simulink model "couple_dmp_test"  (R2020b)
settings: Solver=ode8  StartTime=0.0  StopTime=10.0  FixedStep=0.005  RelTol=1e-3
values from neighbouring files (symbols this model uses):
  Am = [1 8 10]    [my_config_1213.mat]    (also in my_config_1219.mat)
  Bm = [1 10]    [my_config_1213.mat]    (also in my_config_1219.mat)
  cc = [1 0.92774349 0.86070798 0.79851622 0.74081822 0.68728928 0.63762815 0.59155536 0.54881164 0.50915642 0.47236655 0.43823499 ... (41 elements, 1x41)]    [my_config_1213.mat]    (also in my_config_1219.mat)
  D = [64.807 64.807 64.807]    [my_config_1213.mat]    (also in my_config_1219.mat)
  g1 = [-1 0 1]    [my_config_1213.mat]
  g2 = [-1 0.6 1]    [my_config_1213.mat]
  gamma1 = 1.2    [my_config_1213.mat]    (also in my_config_1219.mat)
  gamma2 = 0.5    [my_config_1213.mat]    (also in my_config_1219.mat)
  K = [1050 1050 1050]    [my_config_1213.mat]    (also in my_config_1219.mat; my_config_1224.mat)
  left_0 = [0 0 0]    [my_config_1219.mat]
  m1 = 1    [my_config_1213.mat]    (also in my_config_1219.mat; my_config_1224.mat)
  m2 = 1    [my_config_1213.mat]    (also in my_config_1219.mat; my_config_1224.mat)
  right_0 = [0 0.6 0]    [my_config_1213.mat]    (also in my_config_1219.mat)
  tau1 = 3    [my_config_1213.mat]    (also in my_config_1219.mat)
  weight = [0.0266866854 0.00199886353 0 0.185908993 0.0191898792 0 0.285018336 0.0372844837 0 0.420259935 0.0646488362 0 ... (123 elements, 3x41)]    [my_config_1213.mat]    (also in my_config_1219.mat)
  width = [191.53405062 222.53081866 258.54392519 300.38518553 348.99779456 405.47758835 471.09774681 547.33749391 635.91544276 738.82833688 858.39606128 997.31393782 ... (41 elements, 1x41)]    [my_config_1213.mat]    (also in my_config_1219.mat)
  x1_0 = [0 0.2 0]    [my_config_1213.mat]    (also in my_config_1219.mat; my_config_1224.mat)
  x2_0 = [0 0.4 0]    [my_config_1213.mat]    (also in my_config_1219.mat; my_config_1224.mat)
undefined symbols (not defined in the file or in its folder): b1, b2, b3, k1, k2, k3
settings Model: Creator=10788  LastModifiedBy=10788
settings OptimizationCC: DefaultParameterBehavior=Inlined  UseDivisionForNetSlopeComputation=on  GainParamInheritBuiltInType=on  UseFloatMulNetSlope=on  InlineInvariantSignals=on  PassReuseOutputArgsAs=Individual arguments  ZeroExternalMemoryAtStartup=off  ZeroInternalMemoryAtStartup=off  NoFixptDivByZeroProtection=on  EfficientFloat2IntCast=on  LifeSpan=1  OptimizeBlockOrder=speed  DifferentSizesBufferReuse=on  EfficientTunableParamExpr=on
settings DebuggingCC: ParameterTunabilityLossMsg=error
settings HardwareCC: ProdLongLongMode=on
settings SFSimCC: MATLABDynamicMemAlloc=off  SimTargetLang=C++
settings RTWCC: Description=Embedded Coder  SystemTargetFile=ert.tlc  TemplateMakefile=ert_default_tmf  GenerateReport=on  LaunchReport=on  TargetLang=C++
settings CodeAppCC: ForceParamTrailComments=on  IgnoreCustomStorageClasses=off  OperatorAnnotations=on  SimulinkDataObjDesc=on  SFDataObjDesc=on  CustomSymbolStrGlobalVar=rt$N$M  CustomSymbolStrType=$N$M  CustomSymbolStrFcn=$N$M$F  CustomSymbolStrMacro=$N$M  InsertBlockDesc=on
settings ERTTargetCC: TargetLangStandard=C++03 (ISO)  GenerateSampleERTMain=on  IncludeMdlTerminateFcn=off  CombineSignalStateStructs=on  CodeInterfacePackaging=C++ class  SupportComplex=off  SupportContinuousTime=on  SupportNonInlinedSFcns=on  InlinedParameterPlacement=NonHierarchical  RootIOFormat=Structure reference  ERTCustomFileTemplate=example_file_process.tlc  ERTFilePackagingFormat=CompactWithDataFile

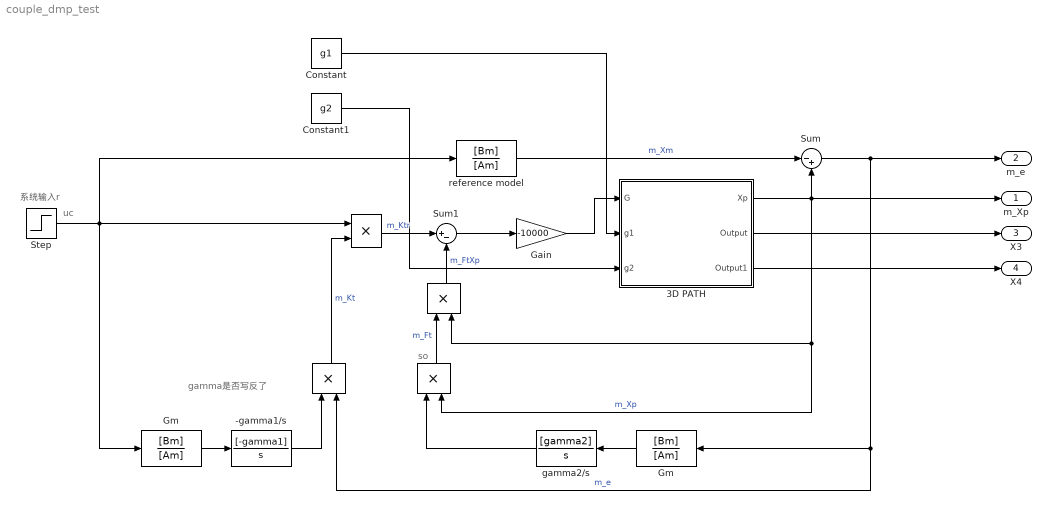
== system couple_dmp_test ==
  note: so
  note: gamma是否写反了
  note: uc
  note: 系统输入r
  " " : Product
  " " : Product
  "  " : Product
  "     " : Product
  -gamma1/s : TransferFcn  Numerator=[-gamma1]  Denominator=[1 0]
  3D PATH : Subsystem
  Constant : Constant  Value=g1
  Constant1 : Constant  Value=g2
  Gain : Gain  Gain=-10000
  "Gm " : TransferFcn  Numerator=[Bm]  Denominator=[Am]
  "Gm  " : TransferFcn  Numerator=[Bm]  Denominator=[Am]
  Step : Step  Time=0  After=0.2  SampleTime=0
  Sum : Sum  Inputs=|-+
  Sum1 : Sum  Inputs=|+-
  gamma2/s : TransferFcn  Numerator=[gamma2]  Denominator=[1 0]
  reference model : TransferFcn  Numerator=[Bm]  Denominator=[Am]
  m_Xp : Outport
  m_e : Outport  Port=2
  X3 : Outport  Port=3
  X4 : Outport  Port=4
  wires:
  "  "/1 -> " "/1  "m_Ft"
  reference model/1 -> Sum/1  "m_Xm"
  gamma2/s/1 -> "  "/1
  "     "/1 -> Sum1/1  "m_Ktr"
  3D PATH/1(Xp) -> "  "/2, " "/2, m_Xp/1, Sum/2  "m_Xp"
  " "/1 -> "     "/2  "m_Kt"
  -gamma1/s/1 -> " "/1
  Gain/1 -> 3D PATH/1(G)
  "Gm  "/1 -> -gamma1/s/1
  Sum1/1 -> Gain/1
  "Gm "/1 -> gamma2/s/1
  Sum/1 -> m_e/1, "Gm "/1, " "/2  "m_e"
  " "/1 -> Sum1/2  "m_FtXp"
  Step/1 -> "Gm  "/1, reference model/1, "     "/1
  3D PATH/2(Output) -> X3/1
  3D PATH/3(Output1) -> X4/1
  Constant/1 -> 3D PATH/2(g1)
  Constant1/1 -> 3D PATH/3(g2)

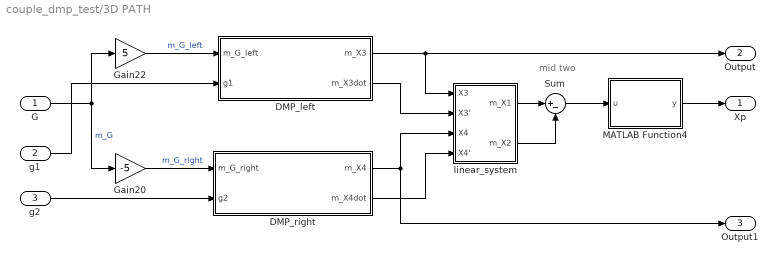
== system couple_dmp_test/3D PATH ==
  note: mid two
  G : Inport
  g1 : Inport  Port=2
  g2 : Inport  Port=3
  DMP_left : Subsystem
  DMP_right : Subsystem
  Gain20 : Gain  Gain=-5
  Gain22 : Gain  Gain=5
  MATLAB Function4 : MATLAB Function  TreatAsAtomicUnit=on
  Sum : Sum  Inputs=|+-
  linear_system : Subsystem
  Xp : Outport
  Output : Outport  Port=2
  Output1 : Outport  Port=3
  wires:
  G/1 -> Gain22/1, Gain20/1  "m_G"
  Sum/1 -> MATLAB Function4/1(u)
  MATLAB Function4/1(y) -> Xp/1
  Gain22/1 -> DMP_left/1(m_G_left)  "m_G_left"
  Gain20/1 -> DMP_right/1(m_G_right)  "m_G_right"
  DMP_left/1(m_X3) -> linear_system/1(X3), Output/1
  DMP_left/2(m_X3dot) -> linear_system/2(X3')
  DMP_right/1(m_X4) -> Output1/1, linear_system/3(X4)
  DMP_right/2(m_X4dot) -> linear_system/4(X4')
  linear_system/1(m_X1) -> Sum/1
  linear_system/2(m_X2) -> Sum/2
  g1/1 -> DMP_left/2(g1)
  g2/1 -> DMP_right/2(g2)

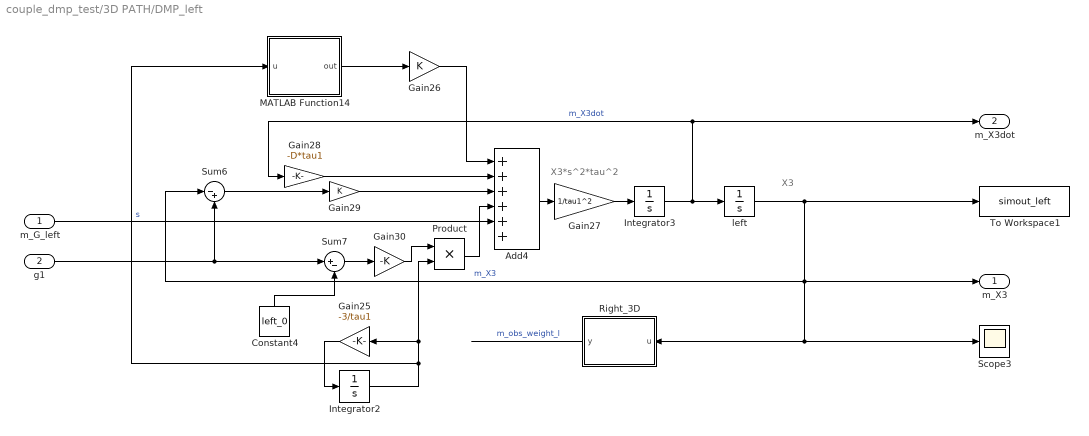
== system couple_dmp_test/3D PATH/DMP_left ==
  note: X3*s^2*tau^2
  note: X3
  m_G_left : Inport
  g1 : Inport  Port=2
  Add4 : Sum  Inputs=++++++
  Constant4 : Constant  Value=left_0
  Gain25 : Gain  Gain=-3/tau1
  Gain26 : Gain  Gain=K
  Gain27 : Gain  Gain=1/tau1^2
  Gain28 : Gain  Gain=-D*tau1
  Gain29 : Gain  Gain=K
  Gain30 : Gain  Gain=-K
  Integrator2 : Integrator  InitialCondition=1
  Integrator3 : Integrator
  MATLAB Function14 : MATLAB Function  TreatAsAtomicUnit=on
  Product : Product
  Right_3D : MATLAB Function  TreatAsAtomicUnit=on
  Scope3 : Scope
  Sum6 : Sum  Inputs=|-+
  Sum7 : Sum  Inputs=|+-
  To Workspace1 : ToWorkspace  VariableName=simout_left  SaveFormat=Timeseries  SampleTime=-1
  left : Integrator  InitialCondition=left_0
  m_X3 : Outport
  m_X3dot : Outport  Port=2
  wires:
  Gain26/1 -> Add4/1
  MATLAB Function14/1(out) -> Gain26/1
  Integrator2/1 -> MATLAB Function14/1(u), Gain25/1, Product/2  "s"
  Sum7/1 -> Gain30/1
  Gain29/1 -> Add4/3
  Gain25/1 -> Integrator2/1
  Gain28/1 -> Add4/2
  Product/1 -> Add4/4
  Gain27/1 -> Integrator3/1
  Sum6/1 -> Gain29/1
  Constant4/1 -> Sum7/2
  Add4/1 -> Gain27/1
  Integrator3/1 -> left/1, m_X3dot/1, Gain28/1  "m_X3dot"
  g1/1 -> Sum7/1, Sum6/2
  left/1 -> Sum6/1, m_X3/1, Right_3D/1(u), Scope3/1, To Workspace1/1  "m_X3"
  Gain30/1 -> Product/1
  m_G_left/1 -> Add4/5
  Right_3D/1(y) -> ?  "m_obs_weight_l"

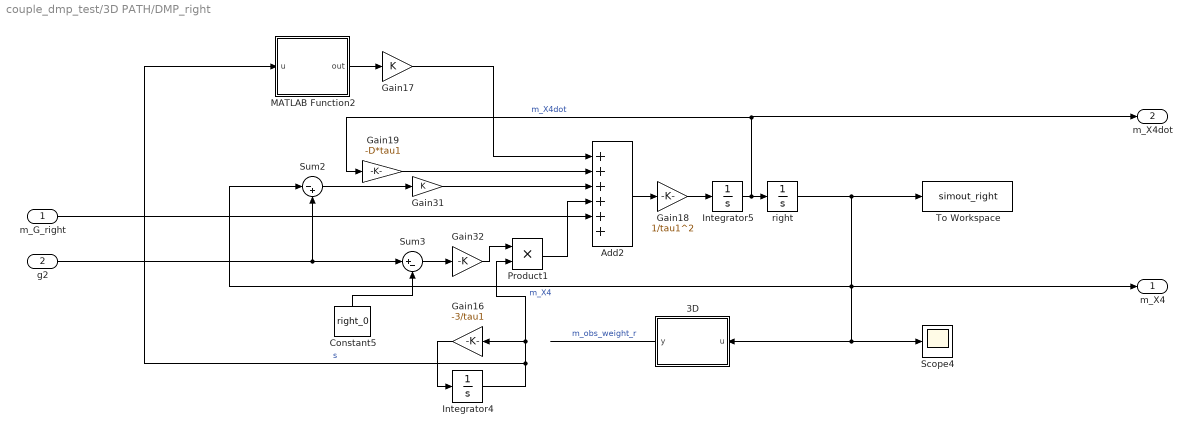
== system couple_dmp_test/3D PATH/DMP_right ==
  m_G_right : Inport
  g2 : Inport  Port=2
  3D : MATLAB Function  TreatAsAtomicUnit=on
  Add2 : Sum  Inputs=++++++
  Constant5 : Constant  Value=right_0
  Gain16 : Gain  Gain=-3/tau1
  Gain17 : Gain  Gain=K
  Gain18 : Gain  Gain=1/tau1^2
  Gain19 : Gain  Gain=-D*tau1
  Gain31 : Gain  Gain=K
  Gain32 : Gain  Gain=-K
  Integrator4 : Integrator  InitialCondition=1
  Integrator5 : Integrator
  MATLAB Function2 : MATLAB Function  TreatAsAtomicUnit=on
  Product1 : Product
  Scope4 : Scope
  Sum2 : Sum  Inputs=|-+
  Sum3 : Sum  Inputs=|+-
  To Workspace : ToWorkspace  VariableName=simout_right  SaveFormat=Timeseries  SampleTime=-1
  right : Integrator  InitialCondition=right_0
  m_X4 : Outport
  m_X4dot : Outport  Port=2
  wires:
  Gain31/1 -> Add2/3
  right/1 -> Sum2/1, m_X4/1, 3D/1(u), Scope4/1, To Workspace/1  "m_X4"
  MATLAB Function2/1(out) -> Gain17/1
  Gain16/1 -> Integrator4/1
  Integrator5/1 -> m_X4dot/1, Gain19/1, right/1  "m_X4dot"
  Sum2/1 -> Gain31/1
  Gain19/1 -> Add2/2
  Constant5/1 -> Sum3/2
  Product1/1 -> Add2/4
  Gain17/1 -> Add2/1
  Integrator4/1 -> Product1/2, Gain16/1, MATLAB Function2/1(u)  "s"
  Sum3/1 -> Gain32/1
  Gain18/1 -> Integrator5/1
  g2/1 -> Sum3/1, Sum2/2
  Add2/1 -> Gain18/1
  Gain32/1 -> Product1/1
  m_G_right/1 -> Add2/5
  3D/1(y) -> ?  "m_obs_weight_r"

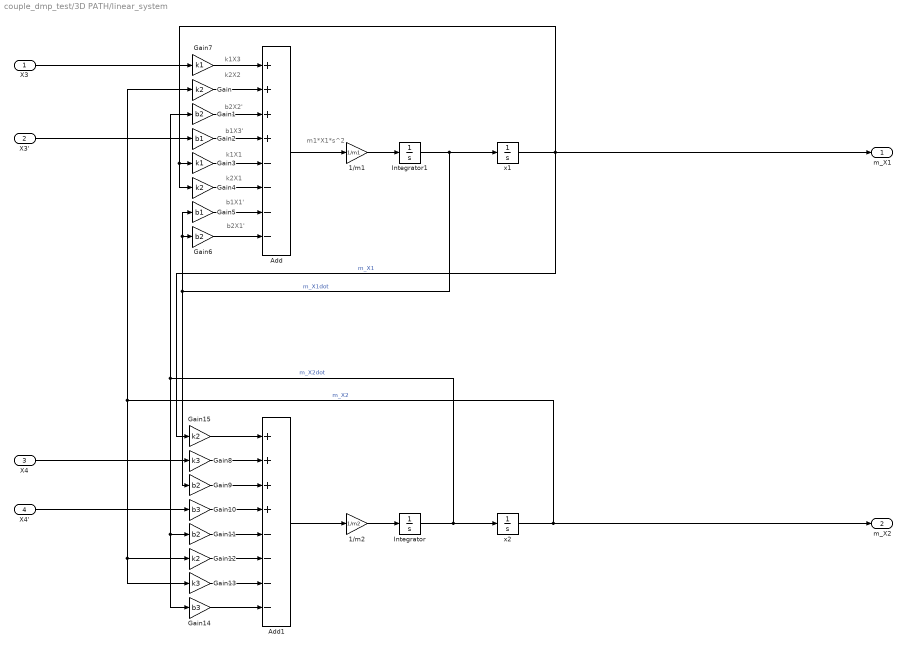
== system couple_dmp_test/3D PATH/linear_system ==
  note: m1*X1*s^2
  note: k1X3
  note: k2X2
  note: b2X2'
  note: b1X3'
  note: k1X1
  note: k2X1
  note: b1X1'
  note: b2X1'
  X3 : Inport
  X3' : Inport  Port=2
  X4 : Inport  Port=3
  X4' : Inport  Port=4
  1/m1 : Gain  Gain=1/m1
  1/m2 : Gain  Gain=1/m2
  Add : Sum  Inputs=++++----
  Add1 : Sum  Inputs=++++----
  Gain{,4,12,15} (4 alike) : Gain  Gain=k2
  Gain{1,6,9,11} (4 alike) : Gain  Gain=b2
  Gain10 : Gain  Gain=b3
  Gain13 : Gain  Gain=k3
  Gain14 : Gain  Gain=b3
  Gain2 : Gain  Gain=b1
  Gain3 : Gain  Gain=k1
  Gain5 : Gain  Gain=b1
  Gain7 : Gain  Gain=k1
  Gain8 : Gain  Gain=k3
  Integrator : Integrator
  Integrator1 : Integrator
  x1 : Integrator  InitialCondition=x1_0
  x2 : Integrator  InitialCondition=x2_0
  m_X1 : Outport
  m_X2 : Outport  Port=2
  wires:
  x1/1 -> Gain15/1, m_X1/1, Gain4/1, Gain3/1  "m_X1"
  Gain7/1 -> Add/1
  Gain3/1 -> Add/5
  1/m1/1 -> Integrator1/1
  Add1/1 -> 1/m2/1
  Gain2/1 -> Add/4
  Gain5/1 -> Add/7
  Gain4/1 -> Add/6
  Gain10/1 -> Add1/4
  X3/1 -> Gain7/1
  Gain6/1 -> Add/8
  Gain1/1 -> Add/3
  Gain15/1 -> Add1/1
  Integrator1/1 -> x1/1, Gain9/1, Gain5/1, Gain6/1  "m_X1dot"
  1/m2/1 -> Integrator/1
  x2/1 -> m_X2/1, Gain/1, Gain13/1, Gain12/1  "m_X2"
  Integrator/1 -> x2/1, Gain1/1, Gain14/1, Gain11/1  "m_X2dot"
  X3'/1 -> Gain2/1
  Add/1 -> 1/m1/1
  Gain/1 -> Add/2
  Gain14/1 -> Add1/8
  Gain13/1 -> Add1/7
  Gain8/1 -> Add1/2
  Gain11/1 -> Add1/5
  X4'/1 -> Gain10/1
  Gain9/1 -> Add1/3
  Gain12/1 -> Add1/6
  X4/1 -> Gain8/1

== matlab function couple_dmp_test/3D PATH/DMP_right/3D ==
  data: u input; y output
function y = fcn(u)

n_dim=3;
n_obt=2;
phi=zeros(n_dim,1);     % 3行1列
phi_tal=zeros(n_dim,1); % 2行1列

% 障碍物1
x_c_1 = 0.2;
y_c_1 = 0.8;
z_c_1 = 0.4;
a_1 = .1;
b_1 = .2;
c_1 = .1;

% 障碍物2
x_c_2 = -0.4;
y_c_2 = 1.2;
z_c_2 = 0.8;
a_2 = 0.15;
b_2 = 0.15;
c_2 = .2;

center=[x_c_1 y_c_1 z_c_1;
    x_c_2 y_c_2 z_c_2
];
axis=[a_1 b_1 c_1;
    a_2 b_2 c_2
];

% center=center(:,[2 1]);
% axis=axis(:,[2 1]);

%%%%%%%%%%%%%

for j=1:n_obt % 障碍物数量
    K = 0;
    for i = 1:n_dim % 坐标维度
        K =K+( (u(i) - center(j,i)) / axis(j,i)) ^2;
    end
    K = K - 1;

    for i = 1:n_dim
        phi(i) = (u(i) - center(j,i)) / axis(j,i) ^2;
    end

    phi = phi * ( exp(-K)) * (1 / K + 1 / K / K) * 2;
    phi_tal=phi_tal+phi;
end

y = phi_tal;

== matlab function couple_dmp_test/3D PATH/DMP_left/MATLAB Function14 ==
  data: u input; out output; width parameter; weight parameter; cc parameter
function out = fcn(u, width, weight, cc)


% if(u>2.5)
%     y=1;
% elseif(u>=0&&u<=2.5)
%     y=0;
% else
%         y=-1;
% end


tem=exp(-width.*(u-cc).^2)';
y=(weight*tem*u)/sum(tem) ;

out = y;

== matlab function couple_dmp_test/3D PATH/DMP_right/MATLAB Function2 ==
  data: u input; out output; width parameter; weight parameter; cc parameter
function out = fcn(u, width, weight, cc)


% if(u>2.5)
%     y=1;
% elseif(u>=0&&u<=2.5)
%     y=0;
% else
%         y=-1;
% end


tem=exp(-width.*(u-cc).^2)';
y=(weight*tem*u)/sum(tem) ;

out = y;

== matlab function couple_dmp_test/3D PATH/MATLAB Function4 ==
  data: u input; y output
function y = fcn(u)

y = norm(u);

== matlab function couple_dmp_test/3D PATH/DMP_left/Right_3D ==
  data: u input; y output
function y = fcn(u)

n_dim=3;
n_obt=1;
phi=zeros(n_dim,1);
phi_tal=zeros(n_dim,1);

x_c_1 = 0.15;
y_c_1 = 0.2;
z_c_1 = 0.4;
a_1 = .1;
b_1 = .1;
c_1 = .1;

x_c_2 = -0.4;
y_c_2 = 1.1;
z_c_2 = 0.8;
a_2 = 0.15;
b_2 = 0.15;
c_2 = .2;

% center=[x_c_1 y_c_1;
%     x_c_2 y_c_2];
% axis=[a_1 b_1;
%     a_2 b_2];

center=[x_c_1 y_c_1 z_c_1;
    x_c_2 y_c_2 z_c_2
];
axis=[a_1 b_1 c_1;
    a_2 b_2 c_2
];

% center=center(:,[2 1]);
% axis=axis(:,[2 1]);

%%%%%%%%%%%%%

for j=1:n_obt
    
    
    K = 0;
for i = 1:n_dim
    
    K =K+( (u(i) - center(j,i)) / axis(j,i)) ^2;
    
end
K = K - 1;

for i = 1:n_dim
    phi(i) = (u(i) - center(j,i)) / axis(j,i) ^2;
   
end

phi =phi * ( exp(-K)) * (1 / K + 1 / K / K) * 2;
      
phi_tal=phi_tal+phi;
end


y = phi_tal;
